simulink model "proyect"  (R2017b)
settings: Solver=ode45  StartTime=0.0  StopTime=15  RelTol=1e-3  EnableMultiTasking=on
settings Model: Creator=Keiver  LastModifiedBy=alfre
settings DataIOCC: LimitDataPoints=on  SaveFormat=Array
settings OptimizationCC: LifeSpan=inf
settings DebuggingCC: SolverPrmCheckMsg=warning  SFUnexpectedBacktrackingDiag=warning  SFNoUnconditionalDefaultTransitionDiag=warning  SFExecutionAtInitializationDiag=none
settings HardwareCC: ProdBitPerPointer=32  ProdBitPerSizeT=32  ProdBitPerPtrDiffT=32  ProdLargestAtomicFloat=None  ProdIntDivRoundTo=Undefined  ProdEndianess=Unspecified  ProdWordSize=32  ProdHWDeviceType=32-bit Generic
settings ModelReferenceCC: PropagateSignalLabelsOutOfModel=off
settings CodeAppCC: StateflowObjectComments=on
settings GRTTargetCC: TargetLangStandard=C89/C90 (ANSI)  GeneratePreprocessorConditionals=Disable all
settings ConfigComp: CovMetricSettings=dw  CovHtmlReporting=on  CovSaveCumulativeToWorkspaceVar=on  CovSaveSingleToWorkspaceVar=on  CovExternalEMLEnable=off  CovSFcnEnable=off

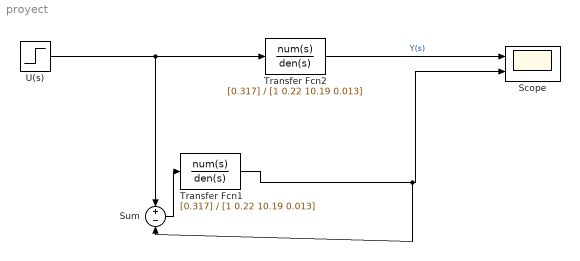
== system proyect ==
  Scope : Scope  NumInputPorts=2
  Sum : Sum  Inputs=+-
  Transfer Fcn1 : TransferFcn  Numerator=[0.317]  Denominator=[1 0.22 10.19 0.013]
  Transfer Fcn2 : TransferFcn  Numerator=[0.317]  Denominator=[1 0.22 10.19 0.013]
  U(s) : Step  Time=0  After=0.8  SampleTime=1
  wires:
  U(s)/1 -> Transfer Fcn2/1, Sum/1
  Transfer Fcn2/1 -> Scope/1  "Y(s)"
  Sum/1 -> Transfer Fcn1/1
  Transfer Fcn1/1 -> Sum/2, Scope/2
